simulink model "BLDC_Controller_Loop"  (R2023b)
settings: Solver=VariableStepAuto  StartTime=0.0  StopTime=10.0  RelTol=1e-3
values from neighbouring files (symbols this model uses):
  SideA_Kt = 0.04189    [ParallelTestBenchParameters.m]
  SideA_N = 7    [ParallelTestBenchParameters.m]
undefined symbols (not defined in the file or in its folder): rad, s
libraries: aerolibconvert2 x1, autolibdatasheetbattery x1, autolibpmsmexterior x1, SignalEditorBlockLib x1, autolibmotorctrlr x1
settings Model: Creator=jwilson  LastModifiedBy=jwilson

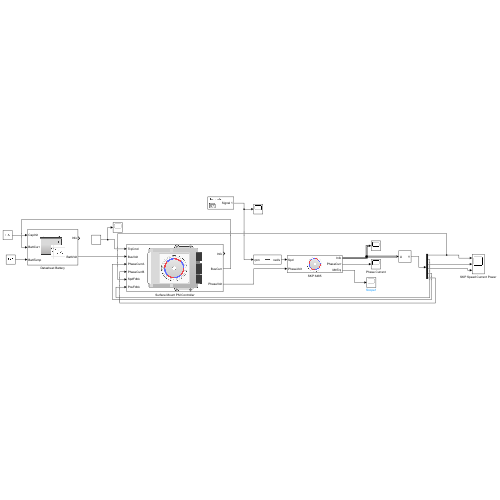
[thumbnail: Simulink's stored preview of the top-level diagram]
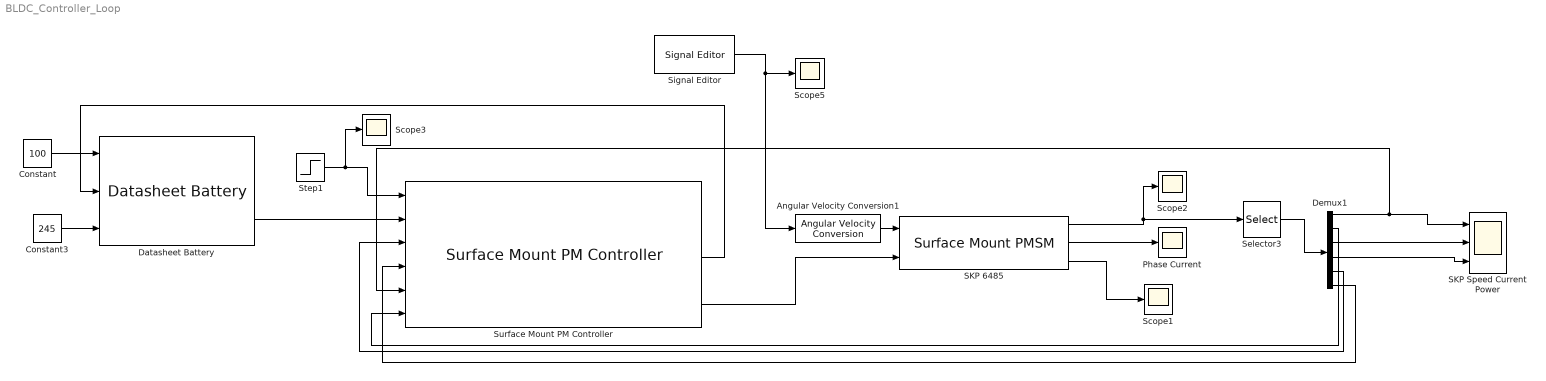
== system BLDC_Controller_Loop ==
  Angular Velocity Conversion1 : aerolibconvert2/Angular Velocity Conversion  IU=rpm  OU=rad/s
  Constant : Constant  Value=100
  Constant3 : Constant  Value=245
  Datasheet Battery : autolibdatasheetbattery/Datasheet Battery  CapacityCtrl=External Input  OutputVlt=Filtered  BattChargeMax=Batt_Cap  Em=[2.8 3.228 3.284 3.361 3.408 3.427 3.472 3.477 3.493 3.504 3.516 3.528 3.537 3.545 3.555 3.561 3.566 3.576 3.587 3.589 3.594 3.6 3.608 3.61 3.616 3.619 3.626 3.632 3.637 3.64 3.645 3.646 3.652 3.655 3.658 3.661 3.664 3.668 3.673 3.678 3.68 3.681 3.686 3.692 3.699 3.702 3.705 3.71 3.717 3.723 3.728 3.733 3.735 3.742 3.749 3.755 3.761 3.768 3.773 3.78 3.791 3.798 3.798 3.814 3.818 3.825 3.841 3.846 3.855 3.863 3.877 3.885 3.894 3.907 3.919 3.926 3.935 3.944 3.954 3.964 3.974 3.988 3.998 4.014 4.029 4.034 4.047 4.065 4.074 4.086 4.097 4.131 4.126 4.138 4.15 4.18 4.174 4.187 4.207 4.231 4.221]  CapLUTBp=[0 0.01 0.02 0.03 0.04 0.05 0.06 0.07 0.08 0.09 0.1 0.11 0.12 0.13 0.14 0.15 0.16 0.17 0.18 0.19 0.2 0.21 0.22 0.23 0.24 0.25 0.26 0.27 0.28 0.29 0.3 0.31 0.32 0.33 0.34 0.35 0.36 0.37 0.38 0.39 0.4 0.41 0.42 0.43 0.44 0.45 0.46 0.47 0.48 0.49 0.5 0.51 0.52 0.53 0.54 0.55 0.56 0.57 0.58 0.59 0.6 0.61 0.62 0.63 0.64 0.65 0.66 0.67 0.68 0.69 0.7 0.71 0.72 0.73 0.74 0.75 0.76 0.77 0.78 0.79 0.8 0.81 0.82 0.83 0.84 0.85 0.86 0.87 0.88 0.89 0.9 0.91 0.92 0.93 0.94 0.95 0.96 0.97 0.98 0.99 1]  RInt=[0.008846 0.009319 0.009027 0.00847 0.01032 0.01314;0.006389 0.006554 0.005553 0.005525 0.006043 0.007805;0.004364 0.004101 0.00406 0.003452 0.003846 0.004517;0.002031 0.002563 0.002532 0.00246 0.002716 0.003047;0.001443 0.001825 0.001795 0.001778 0.001924 0.002234;0.0005603 0.0007192 0.0006887 0.0007557 0.0007355 0.001014;0.001028 0.001338 0.001 0.001536 0.001546 0.002789]  BattTempBp=[243.1 253.1 263.1 273.1 283.1 298.1 313.1]  CapSOCBp=[0 0.2 0.4 0.6 0.8 1]  Ns=Batt_Series  Np=Batt_Parr  BattCapInit=100  Tc=1/1000  Vinit=4.221  RefBlkName='autolibdatasheetbattery/Datasheet Battery'
  Demux1 : Demux  Outputs=6
  Phase Current : Scope
  SKP 6485 : autolibpmsmexterior/Surface Mount PMSM  port_config=Speed  sim_type=Continuous  Ts=0.001  P=SideA_N  Rs=SideA_Rs  Ldq_=SideA_Ldq  KConstText=Permanent flux linkage constant (lambda_pm):  lambda_pm=SideA_lambda  Ke=SideA_Ke  Kt=SideA_Kt  mechanical=SideA_Physical_Param  idq0=[0.5 0.5]  theta_init=0  omega_init=0  KConst=SideA_lambda  lambda_pm_calc=SideA_lambda  RefBlkName='autolibpmsmexterior/Surface Mount PMSM'  aMode=5  Ldq="[0.0017      0.0017]"
  SKP Speed Current Power : Scope  NumInputPorts=3
  Scope{1..3,5} (4 alike) : Scope
  Selector3 : Selector  InputPortWidth=15  IndexOptions=Index vector (dialog)  Indices=[8 9 5 11 1 2]  OutputSizes=1
  Signal Editor : SignalEditorBlockLib/Signal Editor  FileName=Engine Speed Signal.mat  ActiveScenario=Scenario  ActiveSignal=Signal 1  IsBus=off  OutputBusObjectStr=Bus: BusObject  SampleTime=0  ZeroCross=off  OutputAfterFinalValue=Holding final value  Unit=rev/min  PreserveSignalName=on  ApplySigPropsToAllScenarios=on  ApplySigPropsToAllSignals=off
  Step1 : Step  Time=5  After=2  SampleTime=0
  Surface Mount PM Controller : autolibmotorctrlr/Surface Mount PM Controller  control_type=Torque Control  Rs=SideA_Rs  Ldq=SideA_Ldq  Ld=0.000344  Lq=0.000344  lambda_pm=SideA_lambda  PolePairs=SideA_N  Mechanical=SideA_Physical_Param  T_max=SideA_MaxTrq  bp=10  T_mtpa=[0 6.66669841797461 13.3335873347246 20.0008572036754 26.6686983876046 33.3373011134498 40.0068554272732 46.6775511494351 53.3495778300274 60.0231247046184]  id_mtpa=[0 -0.0287202961052195 -0.114874619738106 -0.258443284350566 -0.459393504010068 -0.717679430800711 -1.03324220704656 -1.40601003221657 -1.8358982443354 -2.32280941568585]  iq_mtpa=[0 9.30574388067393 18.6112218818157 27.9161683137524 37.220317866163 46.5234057968387 55.8251681193482 65.12534178925 74.4236648884977 83.7198768076925]  idq_limits=1079.0598  EV_current=200  Tst=5e-5  Kp_d=0.43228  Kp_q=0.43228  Ki=163.3628  EV_motion=[20, 4, 0.8]  EV_sf=200  ba=1.5522  Ksa=39.0064  Kisa=158.1352  Ksf=1217.9727  Jcomp=0.01  Fv=1e-08  Fs=0  param_loss=Single efficiency measurement  eff=98  w_loss_bp=[0 200 400 600 800 1000]  T_loss_bp=[0 25 50 75 100]  losses_table=[100 100 100 100 100;100 150 200 250 300;100 200 300 400 500;100 250 400 550 700;100 300 500 700 900;100 350 600 850 1100]  w_eff_bp=[200 400 600 800 1000]  T_eff_bp=[25 50 75 100]  efficiency_table=[96.2 98.1 98.7 99;98.1 99 99.4 99.5;98.7 99.4 99.6 99.7;99 99.5 99.7 99.8;99.2 99.6 99.7 99.8]  x_w_bp=[-1000 -800 -600 -400 -200 200 400 600 800 1000]  x_T_bp=[-100 -75 -50 -25 25 50 75 100]  x_losses_mat=[200.400801603196 225.67703109328 200.803212851408 201.612903225806 199.999999999997 200 225 200;160.320641282556 180.541624874624 201.005025125625 202.020202020203 200 200 180 160;180.541624874624 180.722891566267 181.086519114686 197.568389057748 194.999999999999 179.999999999997 180 180;201.005025125625 181.086519114686 202.020202020203 193.67991845056 190 200 179.999999999997 200;202.020202020203 197.568389057748 193.67991845056 197.505197505197 190 190 194.999999999999 200;200 194.999999999999 190 190 197.505197505197 193.67991845056 197.568389057748 202.020202020203;200 179.999999999997 200 190 193.67991845056 202.020202020203 181.086519114686 201.005025125625;180 180 179.999999999997 194.999999999999 197.568389057748 181.086519114686 180.722891566267 180.541624874624;160 180 200 200 202.020202020203 201.005025125625 180.541624874624 160.320641282556;200 225 200 199.999999999997 201.612903225806 200.803212851408 225.67703109328 200.400801603196]  Tsm=5e-4
  wires:
  Demux1/1 -> Surface Mount PM Controller/5, SKP Speed Current Power/1
  Demux1/3 -> SKP Speed Current Power/2
  Selector3/1 -> Demux1/1
  Demux1/4 -> SKP Speed Current Power/3
  Surface Mount PM Controller/3 -> SKP 6485/2
  SKP 6485/1 -> Scope2/1, Selector3/1
  SKP 6485/2 -> Phase Current/1
  Demux1/6 -> Surface Mount PM Controller/4
  Demux1/5 -> Surface Mount PM Controller/3
  Demux1/2 -> Surface Mount PM Controller/6
  Datasheet Battery/2 -> Surface Mount PM Controller/2
  Constant3/1 -> Datasheet Battery/3
  Constant/1 -> Datasheet Battery/1
  Surface Mount PM Controller/2 -> Datasheet Battery/2
  SKP 6485/3 -> Scope1/1
  Step1/1 -> Surface Mount PM Controller/1, Scope3/1
  Angular Velocity Conversion1/1 -> SKP 6485/1
  Signal Editor/1 -> Angular Velocity Conversion1/1, Scope5/1
